simulink model "soccerbot"  (R2019b)
settings: Solver=ode15s  StartTime=0.0  StopTime=10.0
PreLoadFcn:
  | addpath(genpath('libraries'));
values from neighbouring files (symbols this model uses):
  plane_dim = [9 6 0.09]    [robotParameters.m]
  start_position = robot.pose.position()    [main.m]    (also in test.m)
undefined symbols (not defined in the file or in its folder): start_configuration, X, Y, Z
libraries: sm_lib x186, nesl_utility x20, Contact_Forces_Lib x8, simulink x1
(part 1 of 4)
settings Model: OrderedModelArguments=off  Creator=robosoccer  LastModifiedBy=vuwij
settings DiagnosticsConfigSet: SimMechanicsRigidlyBoundBlock=none

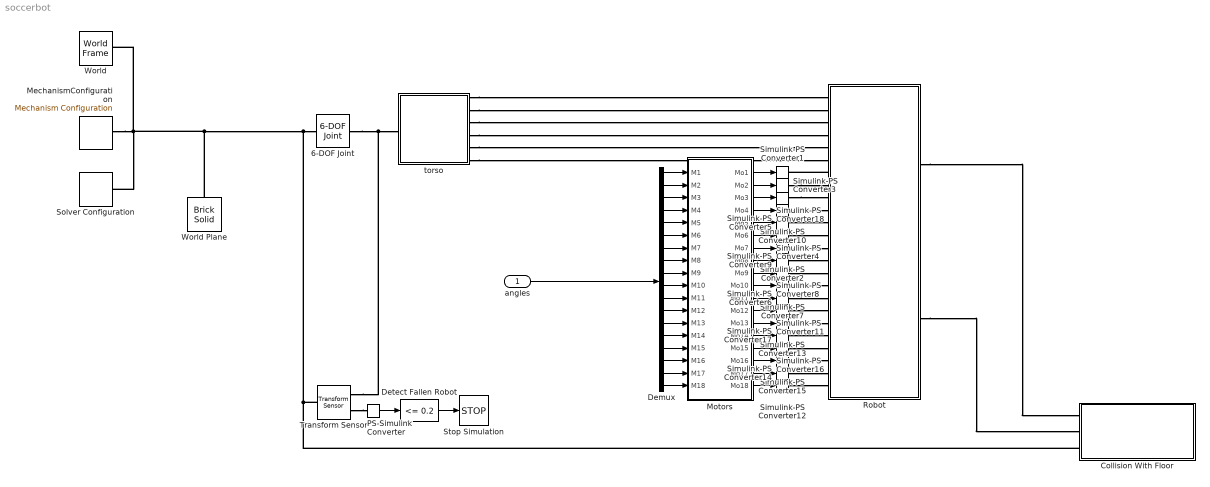
== system soccerbot ==
  angles : Inport
  6-DOF Joint : sm_lib/Joints/6-DOF Joint  JointMode=Normal  SenseConstraintForce=off  SenseConstraintForceX=off  SenseConstraintForceY=off  SenseConstraintForceZ=off  SenseConstraintTorque=off  SenseConstraintTorqueX=off  SenseConstraintTorqueY=off  SenseConstraintTorqueZ=off  SenseTotalForce=off  SenseTotalForceX=off  SenseTotalForceY=off  SenseTotalForceZ=off  SenseTotalTorque=off  SenseTotalTorqueX=off  SenseTotalTorqueY=off  SenseTotalTorqueZ=off  CompositeWrenchDir=FollowerOnBase  CompositeWrenchFrame=BaseFrame  PxEquilibriumPosition=0  PxEquilibriumPositionUnits=m  PxSpringStiffness=0  PxSpringStiffnessUnits=N/m  PxDampingCoefficient=0  PxDampingCoefficientUnits=N/(m/s)  PxTorqueActuationMode=NoTorque  PxMotionActuationMode=ComputedMotion  PxSensePosition=off  PxSenseVelocity=off  PxSenseAcceleration=off  PxSenseTorqueForce=off  PxSenseLowerLimitTorqueForce=off  PxSenseUpperLimitTorqueForce=off  PxLowerLimitSpecify=off  PxLowerLimitBound=-1  PxLowerLimitBoundUnits=m  PxLowerLimitStiffness=1e6  PxLowerLimitStiffnessUnits=N/m  PxLowerLimitDamping=1e3  PxLowerLimitDampingUnits=N/(m/s)  PxLowerLimitTransitionRegionWidth=1e-4  PxLowerLimitTransitionRegionWidthUnits=m  PxUpperLimitSpecify=off  PxUpperLimitBound=1  PxUpperLimitBoundUnits=m  PxUpperLimitStiffness=1e6  PxUpperLimitStiffnessUnits=N/m  PxUpperLimitDamping=1e3  PxUpperLimitDampingUnits=N/(m/s)  PxUpperLimitTransitionRegionWidth=1e-4  PxUpperLimitTransitionRegionWidthUnits=m  PxPositionTargetSpecify=off  PxPositionTargetPriority=High  PxPositionTargetValue=1  PxPositionTargetValueUnits=m  PxVelocityTargetSpecify=off  PxVelocityTargetPriority=High  PxVelocityTargetValue=0  PxVelocityTargetValueUnits=m/s  PyEquilibriumPosition=0  PyEquilibriumPositionUnits=m  PySpringStiffness=0  PySpringStiffnessUnits=N/m  PyDampingCoefficient=0  PyDampingCoefficientUnits=N/(m/s)  PyTorqueActuationMode=NoTorque  PyMotionActuationMode=ComputedMotion  PySensePosition=off  PySenseVelocity=off  PySenseAcceleration=off  PySenseTorqueForce=off  PySenseLowerLimitTorqueForce=off  PySenseUpperLimitTorqueForce=off  PyLowerLimitSpecify=off  PyLowerLimitBound=-1  PyLowerLimitBoundUnits=m  PyLowerLimitStiffness=1e6  PyLowerLimitStiffnessUnits=N/m  PyLowerLimitDamping=1e3  PyLowerLimitDampingUnits=N/(m/s)  PyLowerLimitTransitionRegionWidth=1e-4  PyLowerLimitTransitionRegionWidthUnits=m  PyUpperLimitSpecify=off  PyUpperLimitBound=1  PyUpperLimitBoundUnits=m  PyUpperLimitStiffness=1e6  PyUpperLimitStiffnessUnits=N/m  PyUpperLimitDamping=1e3  PyUpperLimitDampingUnits=N/(m/s)  PyUpperLimitTransitionRegionWidth=1e-4  PyUpperLimitTransitionRegionWidthUnits=m  PyPositionTargetSpecify=off  PyPositionTargetPriority=High  PyPositionTargetValue=0  PyPositionTargetValueUnits=m  PyVelocityTargetSpecify=off  PyVelocityTargetPriority=High  PyVelocityTargetValue=0  PyVelocityTargetValueUnits=m/s  PzEquilibriumPosition=0  PzEquilibriumPositionUnits=m  PzSpringStiffness=0  PzSpringStiffnessUnits=N/m  PzDampingCoefficient=0  PzDampingCoefficientUnits=N/(m/s)  PzTorqueActuationMode=NoTorque  PzMotionActuationMode=ComputedMotion  PzSensePosition=off  PzSenseVelocity=off  PzSenseAcceleration=off  PzSenseTorqueForce=off  PzSenseLowerLimitTorqueForce=off  PzSenseUpperLimitTorqueForce=off  PzLowerLimitSpecify=off  PzLowerLimitBound=-1  PzLowerLimitBoundUnits=m  PzLowerLimitStiffness=1e6  PzLowerLimitStiffnessUnits=N/m  PzLowerLimitDamping=1e3  PzLowerLimitDampingUnits=N/(m/s)  PzLowerLimitTransitionRegionWidth=1e-4  PzLowerLimitTransitionRegionWidthUnits=m  PzUpperLimitSpecify=off  PzUpperLimitBound=1  PzUpperLimitBoundUnits=m  PzUpperLimitStiffness=1e6  PzUpperLimitStiffnessUnits=N/m  PzUpperLimitDamping=1e3  PzUpperLimitDampingUnits=N/(m/s)  PzUpperLimitTransitionRegionWidth=1e-4  PzUpperLimitTransitionRegionWidthUnits=m  PzPositionTargetSpecify=on  PzPositionTargetPriority=High  PzPositionTargetValue=start_position(3) + plane_dim(3)/2  PzPositionTargetValueUnits=m  PzVelocityTargetSpecify=off  PzVelocityTargetPriority=High  PzVelocityTargetValue=0  PzVelocityTargetValueUnits=m/s  SphDefPosRotationMethod=None  SphDefPosRotationAngleUnits=deg  SphDefPosRotationStandardAxis=+Z  SphDefPosRotationAngle=0.0  SphDefPosRotationArbitraryAxis=[0 0 1]  SphDefPosFollAlignAxisA=+X  SphDefPosBaseAlignAxisA=+Y  SphDefPosFollAlignAxisB=+Y  SphDefPosBaseAlignAxisB=+Z  SphDefPosRotationSequenceAxes=FollowerAxes  SphDefPosRotationSequence=XYX  SphDefPosRotationSequenceAngles=[0 0 0]  SphDefPosRotationSequenceAnglesUnits=deg  SphDefPosRotationMatrix=[1 0 0; 0 1 0; 0 0 1]  SphEqPosRotationMethod=None  SphEqPosRotationAngleUnits=deg  SphEqPosRotationStandardAxis=+Z  SphEqPosRotationAngle=0.0  SphEqPosRotationArbitraryAxis=[0 0 1]  SphEqPosFollAlignAxisA=+X  SphEqPosBaseAlignAxisA=+Y  SphEqPosFollAlignAxisB=+Y  SphEqPosBaseAlignAxisB=+Z  SphEqPosRotationSequenceAxes=FollowerAxes  SphEqPosRotationSequence=XYX  SphEqPosRotationSequenceAngles=[0 0 0]  SphEqPosRotationSequenceAnglesUnits=deg  SphEqPosRotationMatrix=[1 0 0; 0 1 0; 0 0 1]  SphSpringStiffness=0  SphSpringStiffnessUnits=N*m/deg  SphDampingCoefficient=0  SphDampingCoefficientUnits=N*m/(deg/s)  SphActuateTorqueX=off  SphActuateTorqueY=off  SphActuateTorqueZ=off  SphActuateTorque=off  SphTorqueActuationMode=NoTorque  SphMotionActuationMode=ComputedMotion  SphActuationFrame=BaseFrame  SphSensePosition=off  SphSenseVelocityX=off  SphSenseVelocityY=off  SphSenseVelocityZ=off  SphSenseVelocity=off  SphSenseAccelerationX=off  SphSenseAccelerationY=off  SphSenseAccelerationZ=off  SphSenseAcceleration=off  SphSenseTorqueX=off  SphSenseTorqueY=off  SphSenseTorqueZ=off  SphSenseTorqueForce=off  SphSenseLowerLimitTorqueMag=off  SphSenseUpperLimitTorqueMag=off  SphSensingFrame=BaseFrame  SphLowerLimitSpecify=off  SphLowerLimitBound=15  SphLowerLimitBoundUnits=deg  SphLowerLimitStiffness=1e4  SphLowerLimitStiffnessUnits=N*m/deg  SphLowerLimitDamping=10  SphLowerLimitDampingUnits=N*m/(deg/s)  SphLowerLimitTransitionRegionWidth=0.1  SphLowerLimitTransitionRegionWidthUnits=deg  SphUpperLimitSpecify=off  SphUpperLimitBound=45  SphUpperLimitBoundUnits=deg  SphUpperLimitStiffness=1e4  SphUpperLimitStiffnessUnits=N*m/deg  SphUpperLimitDamping=10  SphUpperLimitDampingUnits=N*m/(deg/s)  SphUpperLimitTransitionRegionWidth=0.1  SphUpperLimitTransitionRegionWidthUnits=deg  SphPositionTargetRotationMethod=None  SphPositionTargetRotationAngleUnits=deg  SphPositionTargetRotationStandardAxis=+Z  SphPositionTargetRotationAngle=0.0  SphPositionTargetRotationArbitraryAxis=[0 0 1]  SphPositionTargetFollAlignAxisA=+X  SphPositionTargetBaseAlignAxisA=+Y  SphPositionTargetFollAlignAxisB=+Y  SphPositionTargetBaseAlignAxisB=+Z  SphPositionTargetRotationSequenceAxes=FollowerAxes  SphPositionTargetRotationSequence=XYX  SphPositionTargetRotationSequenceAngles=[0 0 0]  SphPositionTargetRotationSequenceAnglesUnits=deg  SphPositionTargetRotationMatrix=[1 0 0; 0 1 0; 0 0 1]  SphPositionTargetSpecify=off  SphPositionTargetPriority=High  SphVelocityTargetValue=[0 0 0]  SphVelocityTargetValueUnits=deg/s  SphVelocityTargetSpecify=off  SphVelocityTargetPriority=High  SphVelocityTargetInFollowerFrame=on
  Collision With Floor : Subsystem
  Demux : Demux  Outputs=18
  Detect Fallen Robot : simulink/Logic and Bit Operations/Compare To Constant  relop=<=  const=0.2  OutDataTypeStr=boolean
  MechanismConfiguration : sm_lib/Utilities/Mechanism Configuration  UniformGravity=Constant  GravityVector=[0 0 -9.80665]  GravityUnits=m/s^2  LinearizationDelta=0.001
  Motors : Subsystem
  PS-Simulink Converter : nesl_utility/PS-Simulink Converter  PhysicalDomain=network_engine_domain  SubClassName=ps_output  LeftPortType=input  RightPortType=output  PseudoPeriodic=off  Frequencies=[]  Unit=inherit  AffineConversion=off
  Robot : Subsystem
  Simulink-PS Converter{1..16} (16 alike) : nesl_utility/Simulink-PS Converter  PhysicalDomain=network_engine_domain  SubClassName=ps_input  LeftPortType=input  RightPortType=output  PseudoPeriodic=off  Frequencies=[]  NoiseDistribution=none  NoiseParameters=[]  Unit=1  AffineConversion=off  FilteringAndDerivatives=filter  SimscapeFilterOrder=2  InputFilterTimeConstant=0.001  UdotUserProvided=0
  Simulink-PS Converter17 : nesl_utility/Simulink-PS Converter  PhysicalDomain=network_engine_domain  SubClassName=ps_input  LeftPortType=input  RightPortType=output  PseudoPeriodic=off  Frequencies=[]  NoiseDistribution=none  NoiseParameters=[]  Unit=1  AffineConversion=off  FilteringAndDerivatives=filter  SimscapeFilterOrder=2  InputFilterTimeConstant=0.001  UdotUserProvided=2
  Simulink-PS Converter18 : nesl_utility/Simulink-PS Converter  PhysicalDomain=network_engine_domain  SubClassName=ps_input  LeftPortType=input  RightPortType=output  PseudoPeriodic=off  Frequencies=[]  NoiseDistribution=none  NoiseParameters=[]  Unit=1  AffineConversion=off  FilteringAndDerivatives=filter  SimscapeFilterOrder=2  InputFilterTimeConstant=0.001  UdotUserProvided=2
  Solver Configuration : nesl_utility/Solver Configuration  PhysicalDomain=network_engine_domain  SubClassName=solver  LeftPortType=input  RightPortType=generic  Tones=[]  Harmonics=[]  SimulateNoise=off  Profile=off  UseLocalSampling=off  EnableSwitchedLinearOptims=on  FrequencyDomain=off  UseCCode=off  RelTol=0.001  AbsTol=1e-06  MinStep=1e-09  ToWorkspace=off  RevertToSquareIcSolve=off  NumHomotopyIterations=100  PhasorMode=off  PhasorModeNumHarmonics=1  DoDC=off  ResidualTolerance=1e-09  UseLocalSolver=off  LocalSolverChoice=NE_BACKWARD_EULER_ADVANCER  LocalSolverSampleTime=0.001  DoFixedCost=off  MaxNonlinIter=3  MaxModeIter=2  LinearAlgebra=auto  EquationFormulation=NE_TIME_EF  DelaysMemoryBudget=1024  AutomaticFiltering=on  FilteringTimeConstant=0.001  PartitionStorageMethod=AS_NEEDED  PartitionMemoryBudget=1024  PartitionMethod=ROBUST
  Stop Simulation : Stop
  Transform Sensor : sm_lib/Frames and Transforms/Transform Sensor  MeasurementFrame=World  SenseAngle=off  SenseAxis=off  SenseAngle1=off  SenseAngle2=off  SenseAngle3=off  SenseQ=off  SenseR=off  SenseOmegaX=off  SenseOmegaY=off  SenseOmegaZ=off  SenseOmega1=off  SenseOmega2=off  SenseOmega3=off  SenseQDot=off  SenseRDot=off  SenseAlphaX=off  SenseAlphaY=off  SenseAlphaZ=off  SenseAlpha1=off  SenseAlpha2=off  SenseAlpha3=off  SenseQDDot=off  SenseRDDot=off  SenseX=off  SenseY=off  SenseZ=on  SenseRad=off  SenseAzim=off  SenseDist=off  SenseInc=off  SenseXDot=off  SenseYDot=off  SenseZDot=off  SenseRadDot=off  SenseAzimDot=off  SenseDistDot=off  SenseIncDot=off  SenseXDDot=off  SenseYDDot=off  SenseZDDot=off  SenseRadDDot=off  SenseAzimDDot=off  SenseDistDDot=off  SenseIncDDot=off
  World : sm_lib/Frames and Transforms/World Frame
  World Plane : sm_lib/Body Elements/Brick Solid  GraphicAmbientColor=[0.15 0.15 0.15 1.0]  BasedOnType=Density  BrickDimensions=plane_dim  BrickDimensionUnits=m  CenterOfMass=[0 0 0]  CenterOfMassUnits=m  GraphicDiffuseColor=[0.0 0.6 0.2]  Density=density  DensityUnits=kg/(m^3)  DoExposeReferenceFrame=on  GraphicEmissiveColor=[0.0 0.0 0.0 1.0]  ExportEntireGeometry=off  SerializedFrames=<Frames/>  MarkerShape=Sphere  MarkerSize=10  GraphicType=FromGeometry  InertiaType=CalculateFromGeometry  Mass=1  MassUnits=kg  MomentsOfInertia=[1 1 1]  MomentsOfInertiaUnits=kg*m^2  GraphicOpacity=0.5  ProductsOfInertia=[0 0 0]  ProductsOfInertiaUnits=kg*m^2  GraphicShininess=75  GraphicSpecularColor=[0.5 0.5 0.5 1.0]  GraphicVisPropType=SimpleVisualProperties
  torso : Subsystem
  wires:
  Detect Fallen Robot/1 -> Stop Simulation/1
  PS-Simulink Converter/1 -> Detect Fallen Robot/1
  angles/1 -> Demux/1
  Demux/2 -> Motors/2(M2)
  Demux/3 -> Motors/3(M3)
  Demux/4 -> Motors/4(M4)
  Demux/5 -> Motors/5(M5)
  Demux/6 -> Motors/6(M6)
  Demux/7 -> Motors/7(M7)
  Demux/8 -> Motors/8(M8)
  Demux/9 -> Motors/9(M9)
  Demux/10 -> Motors/10(M10)
  Demux/11 -> Motors/11(M11)
  Demux/12 -> Motors/12(M12)
  Demux/13 -> Motors/13(M13)
  Demux/14 -> Motors/14(M14)
  Demux/15 -> Motors/15(M15)
  Demux/16 -> Motors/16(M16)
  Demux/17 -> Motors/17(M17)
  Demux/18 -> Motors/18(M18)
  Motors/2(Mo2) -> Simulink-PS Converter3/1
  Motors/3(Mo3) -> Simulink-PS Converter18/1
  Motors/4(Mo4) -> Simulink-PS Converter10/1
  Motors/5(Mo5) -> Simulink-PS Converter5/1
  Motors/6(Mo6) -> Simulink-PS Converter4/1
  Motors/7(Mo7) -> Simulink-PS Converter2/1
  Motors/8(Mo8) -> Simulink-PS Converter9/1
  Motors/9(Mo9) -> Simulink-PS Converter8/1
  Motors/10(Mo10) -> Simulink-PS Converter7/1
  Motors/11(Mo11) -> Simulink-PS Converter6/1
  Motors/12(Mo12) -> Simulink-PS Converter11/1
  Motors/13(Mo13) -> Simulink-PS Converter13/1
  Motors/14(Mo14) -> Simulink-PS Converter17/1
  Motors/15(Mo15) -> Simulink-PS Converter16/1
  Motors/16(Mo16) -> Simulink-PS Converter15/1
  Motors/17(Mo17) -> Simulink-PS Converter14/1
  Motors/18(Mo18) -> Simulink-PS Converter12/1
  Demux/1 -> Motors/1(M1)
  Motors/1(Mo1) -> Simulink-PS Converter1/1
  connections:
  6-DOF Joint/LConn1 -- Transform Sensor/LConn1 -- Collision With Floor/LConn3 -- World Plane/RConn1 -- MechanismConfiguration/RConn1 -- World/RConn1 -- Solver Configuration/RConn1
  6-DOF Joint/RConn1 -- Transform Sensor/RConn1 -- torso/LConn1
  Transform Sensor/RConn2 -- PS-Simulink Converter/LConn1
  torso/RConn1 -- Robot/LConn1
  torso/RConn2 -- Robot/LConn2
  torso/RConn3 -- Robot/LConn3
  torso/RConn4 -- Robot/LConn4
  torso/RConn5 -- Robot/LConn5
  torso/RConn6 -- Robot/LConn6
  Robot/RConn1 -- Collision With Floor/LConn1
  Robot/RConn2 -- Collision With Floor/LConn2
  Robot/LConn7 -- Simulink-PS Converter1/RConn1
  Simulink-PS Converter3/RConn1 -- Robot/LConn8
  Simulink-PS Converter18/RConn1 -- Robot/LConn9
  Simulink-PS Converter10/RConn1 -- Robot/LConn10
  Simulink-PS Converter5/RConn1 -- Robot/LConn11
  Simulink-PS Converter4/RConn1 -- Robot/LConn12
  Simulink-PS Converter2/RConn1 -- Robot/LConn13
  Simulink-PS Converter9/RConn1 -- Robot/LConn14
  Simulink-PS Converter8/RConn1 -- Robot/LConn15
  Simulink-PS Converter7/RConn1 -- Robot/LConn16
  Simulink-PS Converter6/RConn1 -- Robot/LConn17
  Simulink-PS Converter11/RConn1 -- Robot/LConn18
  Simulink-PS Converter13/RConn1 -- Robot/LConn19
  Simulink-PS Converter17/RConn1 -- Robot/LConn20
  Simulink-PS Converter16/RConn1 -- Robot/LConn21
  Simulink-PS Converter15/RConn1 -- Robot/LConn22
  Simulink-PS Converter14/RConn1 -- Robot/LConn23
  Simulink-PS Converter12/RConn1 -- Robot/LConn24

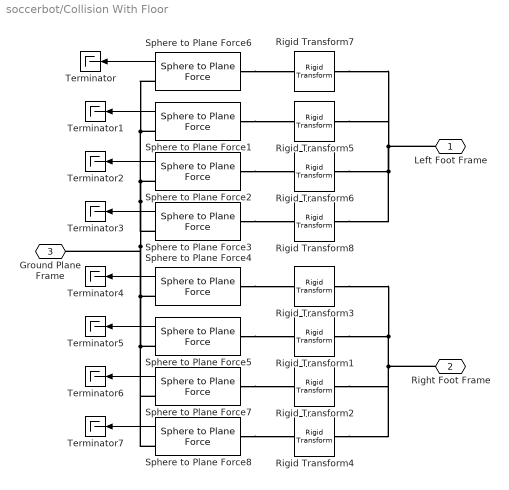
== system soccerbot/Collision With Floor ==
  Rigid Transform1 : sm_lib/Frames and Transforms/Rigid Transform  TranslationMethod=Cartesian  TranslationStandardOffset=0  TranslationLengthUnit=m  TranslationStandardAxis=+Z  TranslationCartesianOffset=left_foot_to_corner_2  TranslationROffset=0  TranslationROffsetUnits=m  TranslationZOffset=0  TranslationZOffsetUnits=m  TranslationThetaOffset=0  TranslationThetaOffsetUnits=deg  RotationMethod=None  RotationAngleUnits=deg  RotationStandardAxis=+Z  RotationAngle=0.0  RotationArbitraryAxis=[0 0 1]  FollAlignAxisA=+X  BaseAlignAxisA=+Y  FollAlignAxisB=+Y  BaseAlignAxisB=+Z  RotationSequenceAxes=FollowerAxes  RotationSequence=XYX  RotationSequenceAngles=[0 0 0]  RotationSequenceAnglesUnits=deg  RotationMatrix=[1 0 0; 0 1 0; 0 0 1]
  Rigid Transform2 : sm_lib/Frames and Transforms/Rigid Transform  TranslationMethod=Cartesian  TranslationStandardOffset=0  TranslationLengthUnit=m  TranslationStandardAxis=+Z  TranslationCartesianOffset=left_foot_to_corner_3  TranslationROffset=0  TranslationROffsetUnits=m  TranslationZOffset=0  TranslationZOffsetUnits=m  TranslationThetaOffset=0  TranslationThetaOffsetUnits=deg  RotationMethod=None  RotationAngleUnits=deg  RotationStandardAxis=+Z  RotationAngle=0.0  RotationArbitraryAxis=[0 0 1]  FollAlignAxisA=+X  BaseAlignAxisA=+Y  FollAlignAxisB=+Y  BaseAlignAxisB=+Z  RotationSequenceAxes=FollowerAxes  RotationSequence=XYX  RotationSequenceAngles=[0 0 0]  RotationSequenceAnglesUnits=deg  RotationMatrix=[1 0 0; 0 1 0; 0 0 1]
  Rigid Transform3 : sm_lib/Frames and Transforms/Rigid Transform  TranslationMethod=Cartesian  TranslationStandardOffset=0  TranslationLengthUnit=m  TranslationStandardAxis=+Z  TranslationCartesianOffset=left_foot_to_corner_1  TranslationROffset=0  TranslationROffsetUnits=m  TranslationZOffset=0  TranslationZOffsetUnits=m  TranslationThetaOffset=0  TranslationThetaOffsetUnits=deg  RotationMethod=None  RotationAngleUnits=deg  RotationStandardAxis=+Z  RotationAngle=0.0  RotationArbitraryAxis=[0 0 1]  FollAlignAxisA=+X  BaseAlignAxisA=+Y  FollAlignAxisB=+Y  BaseAlignAxisB=+Z  RotationSequenceAxes=FollowerAxes  RotationSequence=XYX  RotationSequenceAngles=[0 0 0]  RotationSequenceAnglesUnits=deg  RotationMatrix=[1 0 0; 0 1 0; 0 0 1]
  Rigid Transform4 : sm_lib/Frames and Transforms/Rigid Transform  TranslationMethod=Cartesian  TranslationStandardOffset=0  TranslationLengthUnit=m  TranslationStandardAxis=+Z  TranslationCartesianOffset=left_foot_to_corner_4  TranslationROffset=0  TranslationROffsetUnits=m  TranslationZOffset=0  TranslationZOffsetUnits=m  TranslationThetaOffset=0  TranslationThetaOffsetUnits=deg  RotationMethod=None  RotationAngleUnits=deg  RotationStandardAxis=+Z  RotationAngle=0.0  RotationArbitraryAxis=[0 0 1]  FollAlignAxisA=+X  BaseAlignAxisA=+Y  FollAlignAxisB=+Y  BaseAlignAxisB=+Z  RotationSequenceAxes=FollowerAxes  RotationSequence=XYX  RotationSequenceAngles=[0 0 0]  RotationSequenceAnglesUnits=deg  RotationMatrix=[1 0 0; 0 1 0; 0 0 1]
  Rigid Transform5 : sm_lib/Frames and Transforms/Rigid Transform  TranslationMethod=Cartesian  TranslationStandardOffset=0  TranslationLengthUnit=m  TranslationStandardAxis=+Z  TranslationCartesianOffset=right_foot_to_corner_2  TranslationROffset=0  TranslationROffsetUnits=m  TranslationZOffset=0  TranslationZOffsetUnits=m  TranslationThetaOffset=0  TranslationThetaOffsetUnits=deg  RotationMethod=None  RotationAngleUnits=deg  RotationStandardAxis=+Z  RotationAngle=0.0  RotationArbitraryAxis=[0 0 1]  FollAlignAxisA=+X  BaseAlignAxisA=+Y  FollAlignAxisB=+Y  BaseAlignAxisB=+Z  RotationSequenceAxes=FollowerAxes  RotationSequence=XYX  RotationSequenceAngles=[0 0 0]  RotationSequenceAnglesUnits=deg  RotationMatrix=[1 0 0; 0 1 0; 0 0 1]
  Rigid Transform6 : sm_lib/Frames and Transforms/Rigid Transform  TranslationMethod=Cartesian  TranslationStandardOffset=0  TranslationLengthUnit=m  TranslationStandardAxis=+Z  TranslationCartesianOffset=right_foot_to_corner_3  TranslationROffset=0  TranslationROffsetUnits=m  TranslationZOffset=0  TranslationZOffsetUnits=m  TranslationThetaOffset=0  TranslationThetaOffsetUnits=deg  RotationMethod=None  RotationAngleUnits=deg  RotationStandardAxis=+Z  RotationAngle=0.0  RotationArbitraryAxis=[0 0 1]  FollAlignAxisA=+X  BaseAlignAxisA=+Y  FollAlignAxisB=+Y  BaseAlignAxisB=+Z  RotationSequenceAxes=FollowerAxes  RotationSequence=XYX  RotationSequenceAngles=[0 0 0]  RotationSequenceAnglesUnits=deg  RotationMatrix=[1 0 0; 0 1 0; 0 0 1]
  Rigid Transform7 : sm_lib/Frames and Transforms/Rigid Transform  TranslationMethod=Cartesian  TranslationStandardOffset=0  TranslationLengthUnit=m  TranslationStandardAxis=+Z  TranslationCartesianOffset=right_foot_to_corner_1  TranslationROffset=0  TranslationROffsetUnits=m  TranslationZOffset=0  TranslationZOffsetUnits=m  TranslationThetaOffset=0  TranslationThetaOffsetUnits=deg  RotationMethod=None  RotationAngleUnits=deg  RotationStandardAxis=+Z  RotationAngle=0.0  RotationArbitraryAxis=[0 0 1]  FollAlignAxisA=+X  BaseAlignAxisA=+Y  FollAlignAxisB=+Y  BaseAlignAxisB=+Z  RotationSequenceAxes=FollowerAxes  RotationSequence=XYX  RotationSequenceAngles=[0 0 0]  RotationSequenceAnglesUnits=deg  RotationMatrix=[1 0 0; 0 1 0; 0 0 1]
  Rigid Transform8 : sm_lib/Frames and Transforms/Rigid Transform  TranslationMethod=Cartesian  TranslationStandardOffset=0  TranslationLengthUnit=m  TranslationStandardAxis=+Z  TranslationCartesianOffset=right_foot_to_corner_4  TranslationROffset=0  TranslationROffsetUnits=m  TranslationZOffset=0  TranslationZOffsetUnits=m  TranslationThetaOffset=0  TranslationThetaOffsetUnits=deg  RotationMethod=None  RotationAngleUnits=deg  RotationStandardAxis=+Z  RotationAngle=0.0  RotationArbitraryAxis=[0 0 1]  FollAlignAxisA=+X  BaseAlignAxisA=+Y  FollAlignAxisB=+Y  BaseAlignAxisB=+Z  RotationSequenceAxes=FollowerAxes  RotationSequence=XYX  RotationSequenceAngles=[0 0 0]  RotationSequenceAnglesUnits=deg  RotationMatrix=[1 0 0; 0 1 0; 0 0 1]
  Sphere to Plane Force{1..8} (8 alike) : Contact_Forces_Lib/3D/Sphere to Plane Force  sphere_rad=contact_point_radius  plane_lenx=plane_dim(1)  plane_leny=plane_dim(2)  plane_depth=plane_dim(3)/2  force_law=Linear  k_contact=contact_stiffness  b_contact=contact_damping  pen_full_damp_F=1e-4  pen_exponent=1  custom_param_1=1  custom_param_2=1  friction_law=Stick-Slip Continuous  mu_kinetic=mu_k  mu_static=mu_s  v_thr=mu_vth  vis_on=off  vis_opc_en=0  vis_len_plaBz=0.005  vis_clr=[0.9 0.2 0.2]  vis_opc=0.7
  Terminator{,1..7} (8 alike) : Terminator
  Left Foot Frame : PMIOPort  Side=Left
  Right Foot Frame : PMIOPort  Port=2  Side=Left
  Ground Plane Frame : PMIOPort  Port=3  Side=Left
  wires:
  Sphere to Plane Force6/1 -> Terminator/1
  Sphere to Plane Force8/1 -> Terminator7/1
  Sphere to Plane Force7/1 -> Terminator6/1
  Sphere to Plane Force5/1 -> Terminator5/1
  Sphere to Plane Force4/1 -> Terminator4/1
  Sphere to Plane Force3/1 -> Terminator3/1
  Sphere to Plane Force2/1 -> Terminator2/1
  Sphere to Plane Force1/1 -> Terminator1/1
  connections:
  Sphere to Plane Force8/LConn1 -- Rigid Transform4/RConn1
  Sphere to Plane Force5/LConn1 -- Rigid Transform1/RConn1
  Sphere to Plane Force1/LConn1 -- Rigid Transform5/RConn1
  Rigid Transform4/LConn1 -- Rigid Transform2/LConn1 -- Rigid Transform3/LConn1 -- Rigid Transform1/LConn1 -- Right Foot Frame/RConn1
  Sphere to Plane Force2/LConn1 -- Rigid Transform6/RConn1
  Sphere to Plane Force7/LConn1 -- Rigid Transform2/RConn1
  Sphere to Plane Force4/LConn1 -- Rigid Transform3/RConn1
  Rigid Transform6/LConn1 -- Rigid Transform8/LConn1 -- Left Foot Frame/RConn1 -- Rigid Transform7/LConn1 -- Rigid Transform5/LConn1
  Sphere to Plane Force6/LConn1 -- Rigid Transform7/RConn1
  Sphere to Plane Force2/RConn1 -- Sphere to Plane Force3/RConn1 -- Ground Plane Frame/RConn1 -- Sphere to Plane Force4/RConn1 -- Sphere to Plane Force5/RConn1 -- Sphere to Plane Force8/RConn1 -- Sphere to Plane Force7/RConn1 -- Sphere to Plane Force1/RConn1 -- Sphere to Plane Force6/RConn1
  Sphere to Plane Force3/LConn1 -- Rigid Transform8/RConn1

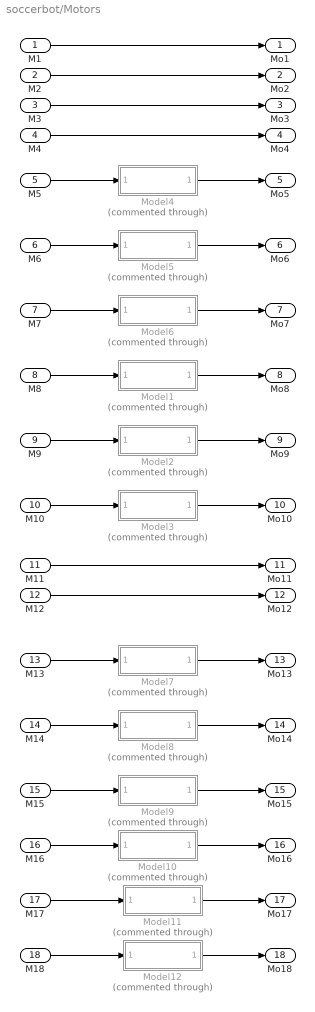
== system soccerbot/Motors ==
  M1 : Inport
  M2 : Inport  Port=2
  M3 : Inport  Port=3
  M4 : Inport  Port=4
  M5 : Inport  Port=5
  M6 : Inport  Port=6
  M7 : Inport  Port=7
  M8 : Inport  Port=8
  M9 : Inport  Port=9
  M10 : Inport  Port=10
  M11 : Inport  Port=11
  M12 : Inport  Port=12
  M13 : Inport  Port=13
  M14 : Inport  Port=14
  M15 : Inport  Port=15
  M16 : Inport  Port=16
  M17 : Inport  Port=17
  M18 : Inport  Port=18
  Model1 : ModelReference  Commented=through  ModelNameDialog=mx28  ParameterArgumentNames=x0  ParameterArgumentValues=start_configuration(8).JointPosition  UsingDefaultArgumentValue=0  SimulationMode=Normal  ModelReferenceVersion=1.33
  Model10 : ModelReference  Commented=through  ModelNameDialog=mx28  ParameterArgumentNames=x0  ParameterArgumentValues=start_configuration(16).JointPosition  UsingDefaultArgumentValue=0  SimulationMode=Normal  ModelReferenceVersion=1.33
  Model11 : ModelReference  Commented=through  ModelNameDialog=mx28  ParameterArgumentNames=x0  ParameterArgumentValues=start_configuration(17).JointPosition  UsingDefaultArgumentValue=0  SimulationMode=Normal  ModelReferenceVersion=1.33
  Model12 : ModelReference  Commented=through  ModelNameDialog=mx28  ParameterArgumentNames=x0  ParameterArgumentValues=start_configuration(18).JointPosition  UsingDefaultArgumentValue=0  SimulationMode=Normal  ModelReferenceVersion=1.33
  Model2 : ModelReference  Commented=through  ModelNameDialog=mx28  ParameterArgumentNames=x0  ParameterArgumentValues=start_configuration(9).JointPosition  UsingDefaultArgumentValue=0  SimulationMode=Normal  ModelReferenceVersion=1.33
  Model3 : ModelReference  Commented=through  ModelNameDialog=mx28  ParameterArgumentNames=x0  ParameterArgumentValues=start_configuration(10).JointPosition  UsingDefaultArgumentValue=0  SimulationMode=Normal  ModelReferenceVersion=1.33
  Model4 : ModelReference  Commented=through  ModelNameDialog=mx28  ParameterArgumentNames=x0  ParameterArgumentValues=start_configuration(5).JointPosition  UsingDefaultArgumentValue=0  SimulationMode=Normal  ModelReferenceVersion=1.33
  Model5 : ModelReference  Commented=through  ModelNameDialog=mx28  ParameterArgumentNames=x0  ParameterArgumentValues=start_configuration(6).JointPosition  UsingDefaultArgumentValue=0  SimulationMode=Normal  ModelReferenceVersion=1.33
  Model6 : ModelReference  Commented=through  ModelNameDialog=mx28  ParameterArgumentNames=x0  ParameterArgumentValues=start_configuration(7).JointPosition  UsingDefaultArgumentValue=0  SimulationMode=Normal  ModelReferenceVersion=1.33
  Model7 : ModelReference  Commented=through  ModelNameDialog=mx28  ParameterArgumentNames=x0  ParameterArgumentValues=start_configuration(13).JointPosition  UsingDefaultArgumentValue=0  SimulationMode=Normal  ModelReferenceVersion=1.33
  Model8 : ModelReference  Commented=through  ModelNameDialog=mx28  ParameterArgumentNames=x0  ParameterArgumentValues=start_configuration(14).JointPosition  UsingDefaultArgumentValue=0  SimulationMode=Normal  ModelReferenceVersion=1.33
  Model9 : ModelReference  Commented=through  ModelNameDialog=mx28  ParameterArgumentNames=x0  ParameterArgumentValues=start_configuration(15).JointPosition  UsingDefaultArgumentValue=0  SimulationMode=Normal  ModelReferenceVersion=1.33
  Mo1 : Outport
  Mo2 : Outport  Port=2
  Mo3 : Outport  Port=3
  Mo4 : Outport  Port=4
  Mo5 : Outport  Port=5
  Mo6 : Outport  Port=6
  Mo7 : Outport  Port=7
  Mo8 : Outport  Port=8
  Mo9 : Outport  Port=9
  Mo10 : Outport  Port=10
  Mo11 : Outport  Port=11
  Mo12 : Outport  Port=12
  Mo13 : Outport  Port=13
  Mo14 : Outport  Port=14
  Mo15 : Outport  Port=15
  Mo16 : Outport  Port=16
  Mo17 : Outport  Port=17
  Mo18 : Outport  Port=18
  wires:
  M5/1 -> Model4/1
  M7/1 -> Model6/1
  M8/1 -> Model1/1
  M9/1 -> Model2/1
  M10/1 -> Model3/1
  M13/1 -> Model7/1
  M14/1 -> Model8/1
  M16/1 -> Model10/1
  M15/1 -> Model9/1
  M1/1 -> Mo1/1
  M2/1 -> Mo2/1
  M3/1 -> Mo3/1
  M4/1 -> Mo4/1
  M11/1 -> Mo11/1
  M12/1 -> Mo12/1
  Model4/1 -> Mo5/1
  Model5/1 -> Mo6/1
  M6/1 -> Model5/1
  Model6/1 -> Mo7/1
  Model1/1 -> Mo8/1
  Model2/1 -> Mo9/1
  Model3/1 -> Mo10/1
  Model7/1 -> Mo13/1
  Model8/1 -> Mo14/1
  Model12/1 -> Mo18/1
  Model11/1 -> Mo17/1
  Model10/1 -> Mo16/1
  Model9/1 -> Mo15/1
  M18/1 -> Model12/1
  M17/1 -> Model11/1
